simulink model "RaptorStateMachine"  (R2018b)
settings: configuration reference "Physics" (kept outside this file)
settings Model: DataDictionary=RaptorStateMachine.sldd  Creator=tobias-ftm  LastModifiedBy=Admin

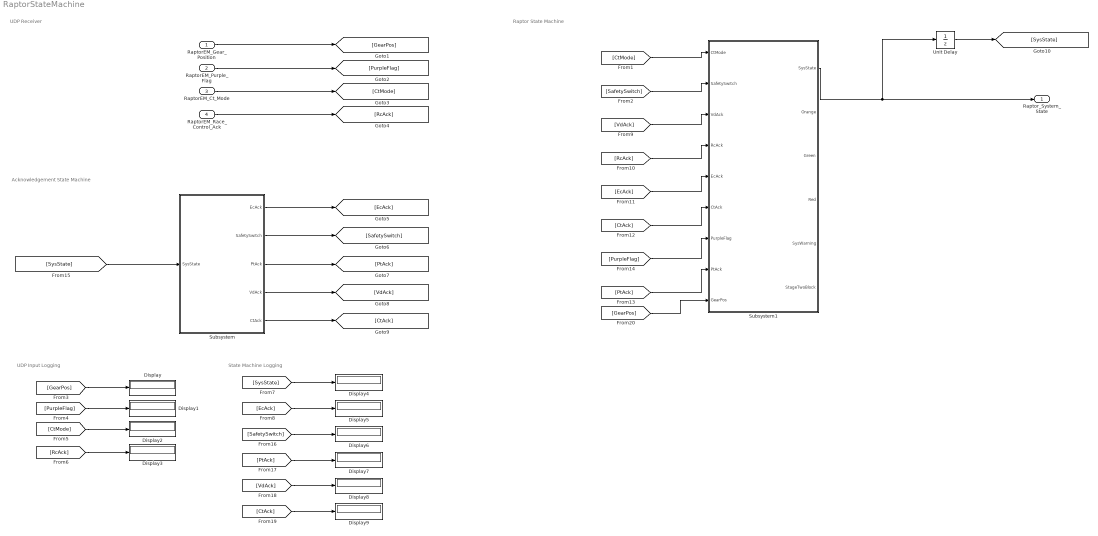
== system RaptorStateMachine ==
  note: Acknowledgement State Machine
  note: Raptor State Machine
  note: UDP Receiver
  note: UDP Input Logging
  note: State Machine Logging
  RaptorEM_Gear_Position : Inport  OutDataTypeStr=uint8
  RaptorEM_Purple_Flag : Inport  Port=2  OutDataTypeStr=uint8
  RaptorEM_Ct_Mode : Inport  Port=3  OutDataTypeStr=uint8
  RaptorEM_Race_Control_Ack : Inport  Port=4  OutDataTypeStr=uint8
  Display{,1..9} (10 alike) : Display
  Subsystem : Subsystem
  Subsystem1 : Subsystem
  Unit Delay : UnitDelay  SampleTime=-1
  Raptor_System_State : Outport
  wires:
  RaptorEM_Gear_Position/1 -> [GearPos]
  RaptorEM_Purple_Flag/1 -> [PurpleFlag]
  RaptorEM_Race_Control_Ack/1 -> [RcAck]
  RaptorEM_Ct_Mode/1 -> [CtMode]
  [GearPos] -> Display/1
  [PurpleFlag] -> Display1/1
  [CtMode] -> Display2/1
  [RcAck] -> Display3/1
  [SysState] -> Display4/1
  [EcAck] -> Display5/1
  [SysState] -> Subsystem/1(SysState)
  Subsystem/1(EcAck) -> [EcAck]
  Subsystem/2(SafetySwitch) -> [SafetySwitch]
  Subsystem/3(PtAck) -> [PtAck]
  Subsystem/4(VdAck) -> [VdAck]
  Subsystem/5(CtAck) -> [CtAck]
  Unit Delay/1 -> [SysState]
  Subsystem1/1(SysState) -> Raptor_System_State/1, Unit Delay/1
  [CtMode] -> Subsystem1/1(CtMode)
  [SafetySwitch] -> Subsystem1/2(SafetySwitch)
  [VdAck] -> Subsystem1/3(VdAck)
  [RcAck] -> Subsystem1/4(RcAck)
  [EcAck] -> Subsystem1/5(EcAck)
  [CtAck] -> Subsystem1/6(CtAck)
  [PurpleFlag] -> Subsystem1/7(PurpleFlag)
  [PtAck] -> Subsystem1/8(PtAck)
  [PtAck] -> Display7/1
  [SafetySwitch] -> Display6/1
  [VdAck] -> Display8/1
  [CtAck] -> Display9/1
  [GearPos] -> Subsystem1/9(GearPos)

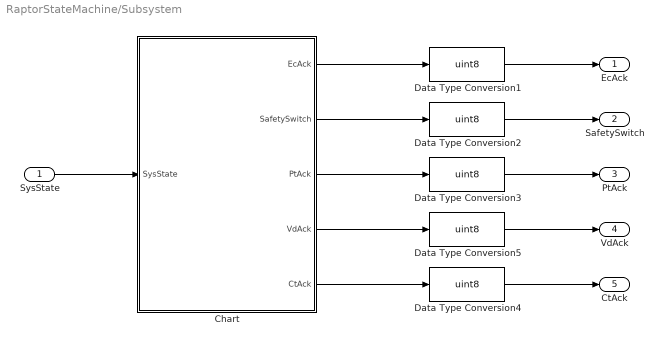
== system RaptorStateMachine/Subsystem ==
  SysState : Inport
  Chart : Stateflow chart  TreatAsAtomicUnit=on
  Data Type Conversion{1..5} (5 alike) : DataTypeConversion  OutDataTypeStr=uint8
  EcAck : Outport
  SafetySwitch : Outport  Port=2
  PtAck : Outport  Port=3
  VdAck : Outport  Port=4
  CtAck : Outport  Port=5
  wires:
  Data Type Conversion1/1 -> EcAck/1
  Data Type Conversion5/1 -> VdAck/1
  Chart/4(VdAck) -> Data Type Conversion5/1
  Data Type Conversion2/1 -> SafetySwitch/1
  Chart/2(SafetySwitch) -> Data Type Conversion2/1
  Chart/1(EcAck) -> Data Type Conversion1/1
  SysState/1 -> Chart/1(SysState)
  Chart/5(CtAck) -> Data Type Conversion4/1
  Data Type Conversion4/1 -> CtAck/1
  Data Type Conversion3/1 -> PtAck/1
  Chart/3(PtAck) -> Data Type Conversion3/1

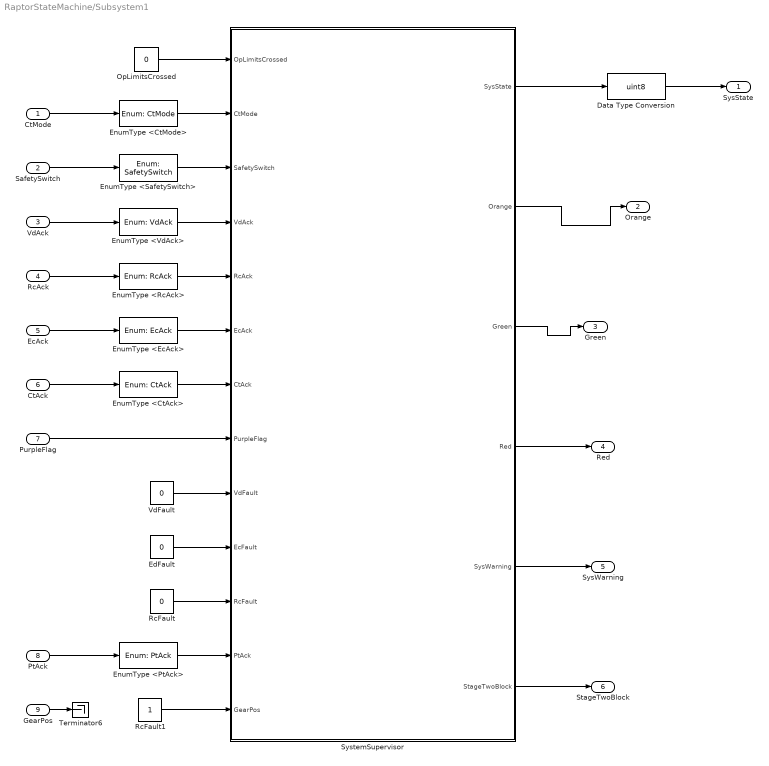
== system RaptorStateMachine/Subsystem1 ==
  CtMode : Inport
  SafetySwitch : Inport  Port=2
  VdAck : Inport  Port=3
  RcAck : Inport  Port=4
  EcAck : Inport  Port=5
  CtAck : Inport  Port=6
  PurpleFlag : Inport  Port=7
  PtAck : Inport  Port=8
  GearPos : Inport  Port=9
  Data Type Conversion : DataTypeConversion  OutDataTypeStr=uint8
  EdFault : Constant  Value=0
  EnumType <CtAck> : DataTypeConversion  OutDataTypeStr=Enum: CtAck
  EnumType <CtMode> : DataTypeConversion  OutDataTypeStr=Enum: CtMode
  EnumType <EcAck> : DataTypeConversion  OutDataTypeStr=Enum: EcAck
  EnumType <PtAck> : DataTypeConversion  OutDataTypeStr=Enum: PtAck
  EnumType <RcAck> : DataTypeConversion  OutDataTypeStr=Enum: RcAck
  EnumType <SafetySwitch> : DataTypeConversion  OutDataTypeStr=Enum: SafetySwitch
  EnumType <VdAck> : DataTypeConversion  OutDataTypeStr=Enum: VdAck
  OpLimitsCrossed : Constant  Value=0  OutDataTypeStr=boolean
  RcFault : Constant  Value=0
  RcFault1 : Constant  OutDataTypeStr=uint8
  SystemSupervisor : Stateflow chart  TreatAsAtomicUnit=on
  Terminator6 : Terminator
  VdFault : Constant  Value=0
  SysState : Outport
  Orange : Outport  Port=2
  Green : Outport  Port=3
  Red : Outport  Port=4
  SysWarning : Outport  Port=5
  StageTwoBlock : Outport  Port=6
  wires:
  EnumType <SafetySwitch>/1 -> SystemSupervisor/3(SafetySwitch)
  OpLimitsCrossed/1 -> SystemSupervisor/1(OpLimitsCrossed)
  EnumType <PtAck>/1 -> SystemSupervisor/12(PtAck)
  EdFault/1 -> SystemSupervisor/10(EcFault)
  RcFault/1 -> SystemSupervisor/11(RcFault)
  SystemSupervisor/5(SysWarning) -> SysWarning/1
  VdAck/1 -> EnumType <VdAck>/1
  EnumType <EcAck>/1 -> SystemSupervisor/6(EcAck)
  SafetySwitch/1 -> EnumType <SafetySwitch>/1
  EnumType <RcAck>/1 -> SystemSupervisor/5(RcAck)
  Data Type Conversion/1 -> SysState/1
  RcAck/1 -> EnumType <RcAck>/1
  CtMode/1 -> EnumType <CtMode>/1
  SystemSupervisor/6(StageTwoBlock) -> StageTwoBlock/1
  SystemSupervisor/4(Red) -> Red/1
  EnumType <CtMode>/1 -> SystemSupervisor/2(CtMode)
  SystemSupervisor/1(SysState) -> Data Type Conversion/1
  EcAck/1 -> EnumType <EcAck>/1
  SystemSupervisor/2(Orange) -> Orange/1
  CtAck/1 -> EnumType <CtAck>/1
  EnumType <VdAck>/1 -> SystemSupervisor/4(VdAck)
  PtAck/1 -> EnumType <PtAck>/1
  PurpleFlag/1 -> SystemSupervisor/8(PurpleFlag)
  VdFault/1 -> SystemSupervisor/9(VdFault)
  EnumType <CtAck>/1 -> SystemSupervisor/7(CtAck)
  RcFault1/1 -> SystemSupervisor/13(GearPos)
  GearPos/1 -> Terminator6/1
  SystemSupervisor/3(Green) -> Green/1

== stateflow chart RaptorStateMachine/Subsystem/Chart ==
  state Default
    EcAck = 2;
    SafetySwitch = 2;
  state PowerOn
    EcAck = 4;
    SafetySwitch = 3;
  state EstablishConnections
    CtAck = 2;
    VdAck = 3;
    PtAck = 3;
  state ActuationTest
    VdAck = 5;
  state ActuationTestPassed
    SafetySwitch = 4;
  state WaitingToCrank
  state CrankChecksInit
    PtAck = 5;
  state CrankChecksPassed
  state EngineStart
    PtAck=7;
  state EngineIdle
  state Driving
  state EmergencyShutdown
    VdAck=12;
    PtAck=11;
  state PowerOff
    VdAck=13;
    EcAck=6;
    SafetySwitch=0;
  state RaptorOff
  (default) -> Default
  Default -> PowerOn : [after(2,sec) && SysState == 1]
  PowerOn -> EstablishConnections : [after(2,sec) && SysState == 2]
  EstablishConnections -> ActuationTest : [after(2,sec)&& SysState == 3]
  ActuationTest -> ActuationTestPassed : [after(2,sec) && SysState == 4]
  ActuationTestPassed -> WaitingToCrank : [after(2,sec) && SysState == 5]
  WaitingToCrank -> CrankChecksInit : [after(2,sec)&&SysState==13]
  CrankChecksInit -> CrankChecksPassed : [after(2,sec) && SysState ==6]
  CrankChecksPassed -> EngineStart : [after(2,sec) && SysState==7]
  EngineStart -> EngineIdle : [after(2,sec)&&SysState==8]
  EngineIdle -> Driving : [after(2,sec)&&SysState==9]
  Driving -> EngineIdle [order 1] : [after(2,sec)&&SysState==8]
  Driving -> EmergencyShutdown [order 2] : [after(2,sec) && SysState==16]
  EmergencyShutdown -> PowerOff : [after(2,sec)&&SysState==11]
  PowerOff -> RaptorOff : [after(2,sec)&&SysState==12]
  data: EcAck output; SafetySwitch output; SysState input; PtAck output; VdAck output; CtAck output

== stateflow chart RaptorStateMachine/Subsystem1/SystemSupervisor ==
  state SystemInit
    state Default
      % Landing state after cartek button is pressed & Safety switch turned to 1
      % IPS, Raptor, MoTeC, SpaceDrive On+Flashing Mode
      % All Ct systems are off
      en: SysWarning = 0; Red=1; Orange = 0; Green =0;
      en,du:
      SysState = SS255_Default;
      if EcFault == 1
      SysWarning = 1; Red=0; Orange = 0; Green =2;
      elseif GearPos ~= 1
      SysWarning = 1; Red=2; Orange = 0; Green =0;
      elseif SafetySwitch == SafetySwitchPosFault
      SysWarning = 1; Red=0; Orange = 2; Green =0;
      else
      Red=1; Orange = 0; Green =0;
      end
      StageTwoBlock = 0;
    state PowerOn
      % All Ct systems powered on
      % Engine off; Veh stationary
      % Ct has no DBW no throttle
      en: SysWarning = 0; Red=1; Orange = 1; Green =0;
      en,du:
      SysState = SS1_PowerOn;
      if EcFault == 2 || SafetySwitch == SafetySwitchPosFault
      SysWarning = 2; Red=1; Orange = 2; Green =0;
      else
      Red=1; Orange = 1; Green =0;
      end
    state EstablishConnections
      % Verify comms with RC and Ct
      % Check Sd, IPS, MoTeC
      % CT has no DBW no throttle
      en: SysWarning = 0; Red=1; Orange = 1; Green =1;
      en,du:
      SysState = SS2_EstConn;
      if VdFault == 1 || RcFault == 1 %Add PtFault condition
      SysWarning = 3; Red=1; Orange = 1; Green =2;
      else
      Red=1; Orange = 1; Green =1;
      end
    Default -> PowerOn : [EcAck == EcAck2_PowerOnStage1Pass &&...
        | SafetySwitch == SafetySwitchPos2 &&...
        | GearPos == 1]
    PowerOn -> EstablishConnections : [CtMode== CtMode2_Initialized && ...
        | EcAck == EcAck4_PowerOnStage2Pass &&...
        | SafetySwitch == SafetySwitchPos3 ]
  note: >>To confirm Raptor sends SD wake command and
      | IPS power-on was successful via current draw and
      | safety switch gets moved from 0 to 1 to indicate
      | "exit low-level controller calibartion mode and power-up
      | 24V systems + GNSS+Radars"
      | >> Don't proceed unless the gear is in neutral
  note: >>CT must check Lidars, cameras, radars & GNSS, and
      | Check current draw confirmation form IPS and
      | safety switch is moved from 1 to 2 to indicate
      | human go-ahead for actuation tests
  note: added this path to enable switching the car off after actuation test success
  state ActuationTestPassed
    en: SysWarning = 0;
    en, du:
    SysState = SS4_ActTestPass;
    % V_Batt check ,Gear oil prs & temp checks
    % Engine oil temp check, Gear pos
    %CT has full DBW, no throttle
    Red=1; Orange = 0; Green =0;
  state ActuationTest
    % Conduct steering, brake test
    % Leak test, actuator limits/response
    % Shift to neutral
    % CT has no DBW no throttle
    en: SysWarning = 0;
    en,du:
    SysState = SS3_ActTest;
    Red=2; Orange = 0; Green =0;
  state CrankChecksInit
    en: SysWarning = 0;
    en,du:
    SysState = SS13_CrankCheckInit;
    Red=1; Orange = 2; Green =0;
  state WaitingToCrank
    en: SysWarning = 0;
    en, du:
    SysState = SS5_WaitToCrank;
    Red=1; Orange = 2; Green =0;
  state ActuationTestFailed
    % Conduct steering, brake test
    % Leak test, actuator limits/response
    % Shift to neutral
    % CT has no DBW no throttle
    en,du:
    SysState = SS14_ActTestFail;
    Red=2; Orange = 2; Green =2;
  note: None(0)
      |     SS255_Default(255)
      |     SS1_PowerOn(1)
      |     SS2_EstConn(2)
      |     SS3_ActTest(3)
      |     SS4_ActTestPass(4)
      |     SS5_WaitToCrank(5)
      |     SS6_CrankChecksPassed(6)
      |     SS7_Crank(7)
      |     SS8_EngineIdle(8)
      |     SS9_Driving(9)
      |     SS10_ShutEngine(10)
      |     SS11_PowerOff(11)
      |     SS12_RaptorOff(12)
      |     SS13_CrankCheckInit(13)
      |     SS14_ActTestFail(14)
      |     SS15_CrankChecksFailed(15)
      |     SS16_EmgShutDown(16)
      |     SS17_EngineFailedToStart(17)
  note: >>Enumeration of VdAck
      |       VdAck0_None
      |       VdAck1_Default
      |       VdAck2_VdEstablishConnectionsAttempt
      |       VdAck3_VdEstablishConnectionsSuccess
      |       VdAck4_ActuationTestAttempt
      |       VdAck5_ActuationTestSuccess
      |       VdAck6_HoldBrakesForCrankOrShutDown
      |       VdAck7_CtSteerBrakeControl
      |       VdAck8_BringToStopSuccess
      |       VdAck9_VDPowerOff
  note: >>Enumeration of RcAck
      | RcAck1_RcFound
      | RcAck2_RcCheckOrangeFlag
      | RcAck3_RcCheckYellowGreenFlag
      | RcAck4_RcMovingChecks
  state NominalOperation
    state CrankChecksPassed
      en: SysWarning = 0;
      % Engine oil temp check, Gear pos
      % CT has no DBW, no throttle
      en,du:
      SysState = SS6_CrankChecksPassed;
      Red=1; Orange = 1; Green =0;
    state CrankChecksFailed
      en: SysWarning = 0;
      en,du:
      SysState = SS15_CrankChecksFailed;
      Red=2; Orange = 2; Green =2;
    state EngineOnline
      state EngineIdle
        % Car may be moving or not
        en,du:
        SysState = SS8_EngineIdle; %6;
        %CT has full DBW no throttle
        %% >> Remove brake & steering control
        Red=1; Orange = 1; Green =2;
      state Driving
        en,du:
        SysState = SS9_Driving;
        %CT has full DBW full throttle
        Red=1; Orange = 1; Green =1;
      EngineIdle -> Driving [order 2] : [CtMode == CtMode7_InitDriving &&...
          |  RcAck == RcAck3_RcCheckYellowGreenFlag]
          | % and VdAck?
      Driving -> EngineIdle : [CtMode == CtMode11_CntrlShudown]
    state EngineStartFailed
      en,du:
      SysState = SS17_EngineFailedToStart;
      Red=2; Orange = 2; Green =2;
    state ShutEngine
      en,du:
      SysState = SS10_ShutEngine; %8;
      %CT has no DBW no throttle
      % Raptor holds brakes (speed scaled?)
      % >> Path to redo actuation tests?
      Red=1; Orange = 1; Green =0;
    state EngineStart
      %Raptor controls crank circ
      %CT has no DBW no throttle
      % Raptor holds brakes (speed scaled?)
      en,du:
      SysState = SS7_Crank;
      Red=1; Orange = 1; Green =2;
    CrankChecksPassed -> (junction 95) [order 2] : [CtMode == CtMode11_CntrlShudown ]
    CrankChecksPassed -> EngineStart [order 1] : [CtMode == CtMode5_StartEngineNow &&...
        |  RcAck == RcAck2_RcCheckOrangeFlag]
    EngineStart -> EngineStartFailed [order 2] : [PtAck == PtAck13_FireEngineFail]
    EngineStart -> EngineIdle [order 1] : [PtAck == PtAck7_FireEngineSuccess]
    EngineIdle -> ShutEngine [order 1] : [CtMode == CtMode11_CntrlShudown]
  note: >>Enumeration of EcAck
      |     EcAck0_None
      |     EcAck1_PowerOnStage1Check
      |     EcAck2_PowerOnStage1Pass
      |     EcAck3_PowerOnStage2Check
      |     EcAck4_PowerOnStage2Pass
      |     EcAck5_PowerOffStage1Check
      |     EcAck6_PowerOffStage1Pass
      |     EcAck7_PowerOffStage2Check
      |     EcAck8_PowerOffStage2Pass
  note: >>CtMode0_Uninitialized(0)
      |       CtMode1_PwrOn(1)
      |       CtMode2_Initialized(2)
      |       CtMode3_ActTest(3)
      |       CtMode4_CrankReady(4)
      |       CtMode5_StartEngineNow(5)
      |       CtMOde6_RaceReady(6)
      |       CtMode7_InitDriving(7)
      |       CtMode8_Caution(8)
      |       CtMode9_NomRace(9)
      |       CtMode10_CoordStop(10)
      |       CtMode11_CntrlShudown(11)
      |       CtMode12_EmrgShutdown(12)
      |       CtMode255_Default(255)
  state CriticalOperatingLimitExceeded
    en,du:
    SS18_CriticalLimitExceeded;
    Red=2; Orange = 2; Green =2;
  state SystemShutdown
    state EmergencyShutdown
      en, du: Red=2; Orange = 2; Green =2;
      SysState = SS16_EmgShutDown;
    state PowerOff
      % SD is turned off % Pretty much everything is off in this state
      en,du:
      SysState = SS11_PowerOff;
      %CT has no DBW no throttle
      Red=1; Orange = 0; Green =0;
    state RaptorOff
      en,du:
      SysState = SS12_RaptorOff;
      Red=0; Orange = 0; Green =0;
    PowerOff -> RaptorOff : [VdAck == VdAck13_VDPowerOffComplete &&...
        |  EcAck == EcAck6_PowerOffStage1Pass &&...
        |   SafetySwitch == SafetySwitchPos0 ]
    EmergencyShutdown -> PowerOff : [VdAck == VdAck12_EmergencyActionsComplete &&...
        | PtAck == PtAck11_EngineOffSuccesful]
  (default) -> Default
  (junction 116) -> (junction 114)
  (junction 114) -> PowerOff
  ActuationTestPassed -> (junction 116) [order 2] : [CtMode == CtMode11_CntrlShudown]
  EstablishConnections -> ActuationTest : [after(5,sec) && CtAck == CtAck2_CtOnline &&...
      | VdAck == VdAck3_VdEstablishConnectionsSuccess &&...
      | RcAck == RcAck1_RcFound && ...
      | PtAck == PtAck3_PtEstablishConnectionsSuccess]
  ActuationTest -> ActuationTestPassed [order 1] : [VdAck == VdAck5_ActuationTestSuccess]
  ActuationTestPassed -> WaitingToCrank [order 1] : [ SafetySwitch == SafetySwitchPos4 ]
  ActuationTest -> ActuationTestFailed [order 2] : [VdAck == VdAck10_ActuationTestFail]
  SystemInit -> (junction 193) : [SafetySwitch == SafetySwitchPos0 && after(5,sec)]
  WaitingToCrank -> CrankChecksInit : [CtMode == CtMode4_CrankReady && ...
      | after(30,sec)]
  CrankChecksInit -> CrankChecksFailed [order 2] : [PtAck == PtAck12_PtPreCrankCheckFail]
  CrankChecksInit -> CrankChecksPassed [order 1] : [PtAck == PtAck5_PtPreCrankCheckSuccess]
  ActuationTestFailed -> (junction 168) : [after(10,sec)]
  (junction 95) -> PowerOff
  CrankChecksFailed -> (junction 168) : [after(10,sec)]
  (junction 168) -> (junction 179)
  EngineStartFailed -> (junction 179) : [after(10,sec)]
  (junction 179) -> (junction 160)
  ShutEngine -> PowerOff : [PtAck == PtAck11_EngineOffSuccesful]
  EngineOnline -> CriticalOperatingLimitExceeded : [OpLimitsCrossed == 1]
  NominalOperation -> EmergencyShutdown : [PurpleFlag == 1 || CtAck == CtAck3_CtControlSuspended || ...
      | CtMode == CtMode12_EmrgShutdown]
  CriticalOperatingLimitExceeded -> EmergencyShutdown : [after(2,sec)]
  (junction 193) -> (junction 160) : {StageTwoBlock = 1;}
  (junction 160) -> PowerOff
  data: OpLimitsCrossed input boolean; CtMode input Enum: CtMode; SafetySwitch input Enum: SafetySwitch; VdAck input Enum: VdAck; SysState output Enum: SystemStates; RcAck input Enum: RcAck; EcAck input Enum: EcAck; CtAck input Enum: CtAck; PurpleFlag input; Orange output uint8 size=1; Green output uint8 size=1; Red output uint8 size=1; SysWarning output uint8 size=1; VdFault input; EcFault input; RcFault input; PtAck input Enum: PtAck; GearPos input; StageTwoBlock output size=1
